simulink model "PQ_Control_LCL"  (R2023b)
settings: Solver=FixedStepAuto  StartTime=0.0  StopTime=10.0  RelTol=1e-3
InitFcn:
  | Initialization_for_PQ_Control_LCL;
values from neighbouring files (symbols this model uses):
  Fnom_Grid = 50    [Initialization_for_PQ_Control_LCL.m]
  Gain_for_ActiveDamping = 0.8    [VariablesDictionary_for_PQ_Control_LCL.sldd]
  Inom = Pnom/sqrt(3)/Unom_Grid    [Initialization_for_PQ_Control_LCL.m]
  Ki_Idq = Kp_Idq*2*pi*10    (= 157.913670417)    [Initialization_for_PQ_Control_LCL.m]
  Kp_Idq = L_grid*2*pi*2000    (= 2.51327412287)    [Initialization_for_PQ_Control_LCL.m]
  L_grid = 200e-6    (= 0.0002)    [Initialization_for_PQ_Control_LCL.m]
  Pnom = 220e3    (= 220000)    [Initialization_for_PQ_Control_LCL.m]
  Ts_Control = 62.5e-6    (= 6.25e-05)    [Initialization_for_PQ_Control_LCL.m]
  Udc_ref = 1500    [Initialization_for_PQ_Control_LCL.m]
  Unom_Phase = Unom_Grid/sqrt(3)    [Initialization_for_PQ_Control_LCL.m]
  Wp_compensation = 148.99    [VariablesDictionary_for_PQ_Control_LCL.sldd]
  Wz_compensation = 314.1592    [VariablesDictionary_for_PQ_Control_LCL.sldd]
libraries: LibraryForCodeGeneration x12
settings Model: DataDictionary=VariablesDictionary_for_PQ_Control_LCL.sldd  TunableVars=Inom,Ki_Idq,Kp_Idq,Udc_ref,Unom_Phase  TunableVarsStorageClass=Auto,Auto,Auto,Auto,Auto  TunableVarsTypeQualifier=,,,,  Creator=ZZY  LastModifiedBy=y
settings OptimizationCC: BlockReduction=off  DefaultParameterBehavior=Inlined  UseDivisionForNetSlopeComputation=on  DefaultUnderspecifiedDataType=single  ReuseModelBlockBuffer=off  ExpressionFolding=off  PassReuseOutputArgsAs=Individual arguments  ZeroExternalMemoryAtStartup=off  ZeroInternalMemoryAtStartup=off  EfficientFloat2IntCast=on  LifeSpan=inf  OptimizationLevel=level1  LabelGuidedReuse=on  EfficientTunableParamExpr=on
settings DebuggingCC: SignalInfNanChecking=warning  SignalRangeChecking=warning  ReadBeforeWriteMsg=EnableAllAsError  WriteAfterWriteMsg=EnableAllAsError  WriteAfterReadMsg=EnableAllAsError  IntegerOverflowMsg=error  ParameterPrecisionLossMsg=none  FixptConstUnderflowMsg=warning  FixptConstOverflowMsg=warning  FixptConstPrecisionLossMsg=warning  UnnecessaryDatatypeConvMsg=warning  UniqueDataStoreMsg=error  AssertControl=DisableAll  NonBusSignalsTreatedAsBus=error  SFInvalidInputDataAccessInChartInitDiag=error  SFTransitionOutsideNaturalParentDiag=error  SFUnreachableExecutionPathDiag=error  SFUndirectedBroadcastEventsDiag=error  IntegerSaturationMsg=error
settings HardwareCC: ProdBitPerChar=16  ProdBitPerInt=16  ProdBitPerPointer=32  ProdBitPerSizeT=32  ProdBitPerPtrDiffT=32  ProdLargestAtomicInteger=Integer  ProdLargestAtomicFloat=None  ProdWordSize=16  ProdHWDeviceType=Texas Instruments->C2000  TargetBitPerChar=16  TargetBitPerInt=16  TargetLargestAtomicInteger=Integer  TargetIntDivRoundTo=Zero  TargetEndianess=LittleEndian  TargetWordSize=16  TargetHWDeviceType=Texas Instruments->C2000
settings SFSimCC: CompileTimeRecursionLimit=0  EnableRuntimeRecursion=off  MATLABDynamicMemAlloc=off
settings RTWCC: Description=Embedded Coder  SystemTargetFile=ert.tlc  TemplateMakefile=ert_default_tmf  GenerateReport=on  Toolchain=MinGW64 | gmake (64-bit Windows)  BuildConfiguration=Faster Runs  IncludeHyperlinkInReport=on  LaunchReport=on  DataTypeReplacement=CDataTypesFixedWidth  GenerateTraceInfo=on  GenerateTraceReport=on  GenerateTraceReportSl=on  GenerateTraceReportSf=on  GenerateTraceReportEml=on  GenerateWebview=on  GenerateCodeReplacementReport=on  CheckMdlBeforeBuild=Warning
settings CodeAppCC: ForceParamTrailComments=on  IgnoreCustomStorageClasses=off  OperatorAnnotations=on  SimulinkDataObjDesc=on  SFDataObjDesc=on  MATLABFcnDesc=on  DefineNamingRule=UpperCase  InsertBlockDesc=on  StateflowObjectComments=on  MATLABSourceComments=on  InlinedPrmAccess=Macros  ReqsInCode=on
settings ERTTargetCC: TargetLangStandard=C99 (ISO)  GenerateSampleERTMain=on  CombineSignalStateStructs=on  GroupInternalDataByFunction=on  ParenthesesLevel=Standards  CastingMode=Standards  GenerateSharedConstants=off  ERTCustomFileTemplate=example_file_process.tlc  RateTransitionBlockCode=Function  PreserveExpressionOrder=on  PreserveIfCondition=on  ConvertIfToSwitch=off  SuppressUnreachableDefaultCases=off  EnableSignedLeftShifts=off  EnableSignedRightShifts=off  MaxIdInt64=INT64_MAX  MinIdInt64=INT64_MIN  MaxIdUint64=UINT64_MAX  MaxIdInt32=INT32_MAX  MinIdInt32=INT32_MIN  MaxIdUint32=UINT32_MAX  MaxIdInt16=INT16_MAX  MinIdInt16=INT16_MIN  MaxIdUint16=UINT16_MAX  MaxIdInt8=INT8_MAX  MinIdInt8=INT8_MIN  MaxIdUint8=UINT8_MAX

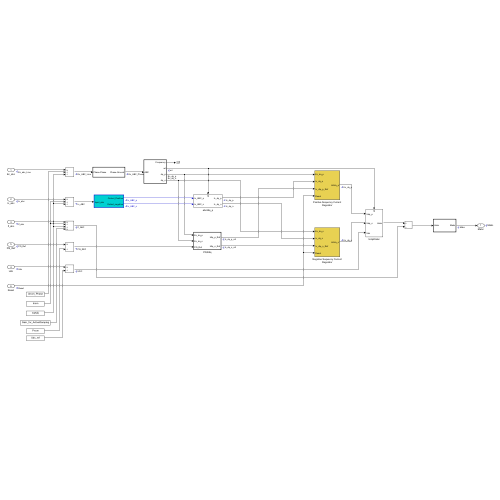
[thumbnail: Simulink's stored preview of the top-level diagram]
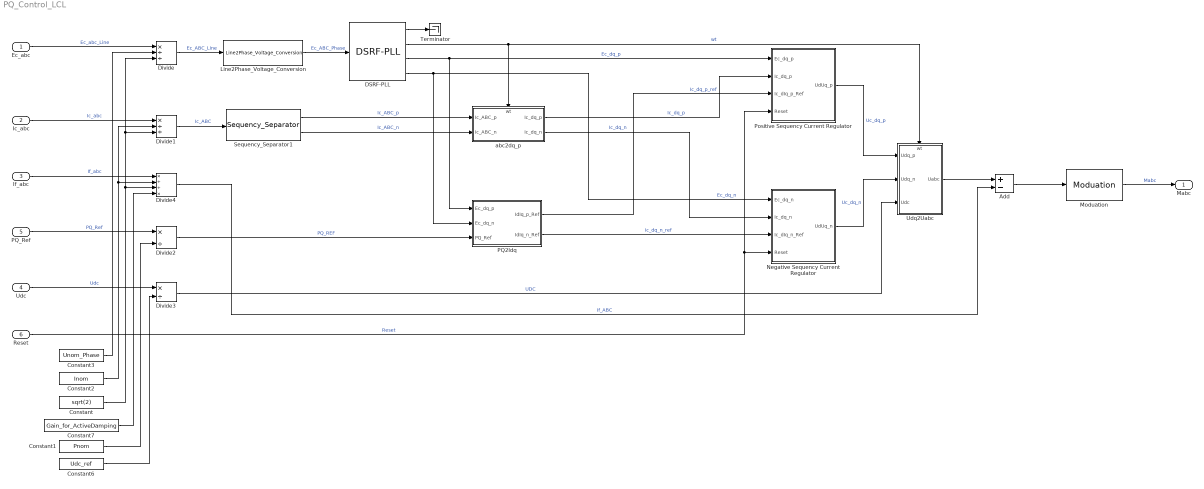
== system PQ_Control_LCL ==
  Ec_abc : Inport  OutDataTypeStr=single  PortDimensions=3
  Ic_abc : Inport  Port=2  OutDataTypeStr=single  PortDimensions=3
  If_abc : Inport  Port=3  OutDataTypeStr=single  PortDimensions=3
  Udc : Inport  Port=4  OutDataTypeStr=single
  PQ_Ref : Inport  Port=5  OutDataTypeStr=single
  Reset : Inport  Port=6  OutDataTypeStr=boolean
  Add : Sum  Inputs=+-
  Constant : Constant  Value=sqrt(2)  OutDataTypeStr=Inherit: Inherit via back propagation  SampleTime=-1
  Constant1 : Constant  Value=Pnom  OutDataTypeStr=Inherit: Inherit via back propagation  SampleTime=-1
  Constant2 : Constant  Value=Inom  OutDataTypeStr=Inherit: Inherit via back propagation  SampleTime=-1
  Constant3 : Constant  Value=Unom_Phase  OutDataTypeStr=Inherit: Inherit via back propagation  SampleTime=-1
  Constant6 : Constant  Value=Udc_ref  OutDataTypeStr=Inherit: Inherit via back propagation  SampleTime=-1
  Constant7 : Constant  Value=Gain_for_ActiveDamping  OutDataTypeStr=Inherit: Inherit via back propagation  SampleTime=-1
  DSRF-PLL : LibraryForCodeGeneration/DSRF-PLL  Ts=Ts_Control  Wc=2*pi*50*0.707  Wf=2*pi*50  Kp=2*pi*25*2*0.707  Ki=power(2*pi*25,2)
  Divide : Product  Inputs=*//  OutDataTypeStr=single
  Divide1 : Product  Inputs=*//  OutDataTypeStr=single
  Divide2 : Product  Inputs=*/  OutDataTypeStr=single
  Divide3 : Product  Inputs=*/  OutDataTypeStr=single
  Divide4 : Product  Inputs=*//*  OutDataTypeStr=single
  Line2Phase_Voltage_Conversion : LibraryForCodeGeneration/Line2Phase_Voltage_Conversion  SystemSampleTime=-1  VariantActivationTime=update diagram  AllowFlexibleInterface=on  Latency=0  AutoFrameSizeCalculation=off
  Moduation : LibraryForCodeGeneration/Moduation  Modulation=Modulation
  Negative Sequency Current Regulator : Subsystem
  PQ2Idq : Subsystem  TreatAsAtomicUnit=on
  Positive Sequency Current Regulator : Subsystem
  Sequency_Separator1 : LibraryForCodeGeneration/Sequency_Separator  SystemSampleTime=-1  VariantActivationTime=update diagram  AllowFlexibleInterface=on  Latency=0  AutoFrameSizeCalculation=off
  Terminator : Terminator
  Udq2Uabc : Subsystem
      settings: PortSchema="{\"entries\":[{\"content\":{\"sides\":[{\"content\":{\"connectorIds\":[\"In1\",\"In2\",\"In3\"]},\"type\":\"ConnectorPlacement.EquallySpacedRectSide\",\"uuid\":\"009786f4-728c-4160-b9bf-eaf0b5a05101\"},{\"content\":{\"connectorIds\":[\"Out1\"],\"side\":\"RIGHT\"},\"type\":\"ConnectorPlacement.EquallySpacedRectSide\",\"uuid\":\"2a94367a-5c57-4632-9573-ab089470159a\"},{\"content\":{\"connectorIds\":[\"In4\"],\"side\":\"TOP\"},\"type\":\"ConnectorPlacement.EquallySpacedRectSide\",\"uuid\":\"6906365b-3187-4c4b-97cf-c9dec4c5ef7c\"}]},\"type\":\"ConnectorPlacement.EquallySpacedConnector\",\"uuid\":\"96ca8566-a266-405c-817a-b47b433d51ed\"}],\"packageUris\":[\"http://schema.mathworks.com/mf0/Connector/R2020b\"],\"version\":\"1.0\"}"
  abc2dq_p : Subsystem
      settings: PortSchema="{\"entries\":[{\"content\":{\"sides\":[{\"content\":{\"connectorIds\":[\"In1\",\"In2\"]},\"type\":\"ConnectorPlacement.EquallySpacedRectSide\",\"uuid\":\"702c7fae-dbbb-427d-af19-afd468018ae6\"},{\"content\":{\"connectorIds\":[\"Out1\",\"Out2\"],\"side\":\"RIGHT\"},\"type\":\"ConnectorPlacement.EquallySpacedRectSide\",\"uuid\":\"d2ca5462-a446-46d8-bb73-1a455ffa959f\"},{\"content\":{\"connectorIds\":[\"In3\"],\"side\":\"TOP\"},\"type\":\"ConnectorPlacement.EquallySpacedRectSide\",\"uuid\":\"50bc6c44-424f-4342-960e-11540364fe97\"}]},\"type\":\"ConnectorPlacement.EquallySpacedConnector\",\"uuid\":\"f58cf64d-fe35-43f1-a031-7ee625a8bb1e\"}],\"packageUris\":[\"http://schema.mathworks.com/mf0/Connector/R2020b\"],\"version\":\"1.0\"}"
  Mabc : Outport  SignalName=Mabc  OutDataTypeStr=single  PortDimensions=3
      settings: MustResolveToSignalObject=on
  wires:
  Line2Phase_Voltage_Conversion/1 -> DSRF-PLL/1  "Ec_ABC_Phase"
  Divide2/1 -> PQ2Idq/3(PQ_Ref)  "PQ_REF"
  PQ_Ref/1 -> Divide2/1  "PQ_Ref"
  PQ2Idq/1(IdIq_p_Ref) -> Positive Sequency Current Regulator/3(Ic_dIq_p_Ref)  "Ic_dq_p_ref"
  abc2dq_p/2(Ic_dq_n) -> Negative Sequency Current Regulator/2(Ic_dq_n)  "Ic_dq_n"
  Positive Sequency Current Regulator/1(UdUq_p) -> Udq2Uabc/1(Udq_p)  "Uc_dq_p"
  Divide3/1 -> Udq2Uabc/3(Udc)  "UDC"
  DSRF-PLL/3 -> Positive Sequency Current Regulator/1(Ec_dq_p), PQ2Idq/1(Ec_dq_p)  "Ec_dq_p"
  Ec_abc/1 -> Divide/1  "Ec_abc_Line"
  abc2dq_p/1(Ic_dq_p) -> Positive Sequency Current Regulator/2(Ic_dq_p)  "Ic_dq_p"
  Divide1/1 -> Sequency_Separator1/1  "Ic_ABC"
  Ic_abc/1 -> Divide1/1  "Ic_abc"
  DSRF-PLL/4 -> Negative Sequency Current Regulator/1(Ec_dq_n), PQ2Idq/2(Ec_dq_n)  "Ec_dq_n"
  Divide/1 -> Line2Phase_Voltage_Conversion/1  "Ec_ABC_Line"
  Udc/1 -> Divide3/1  "Udc"
  PQ2Idq/2(IdIq_n_Ref) -> Negative Sequency Current Regulator/3(Ic_dIq_n_Ref)  "Ic_dq_n_ref"
  Constant3/1 -> Divide/2
  Constant/1 -> Divide4/3, Divide1/3, Divide/3
  Constant2/1 -> Divide4/2, Divide1/2
  Constant6/1 -> Divide3/2
  Reset/1 -> Positive Sequency Current Regulator/4(Reset), Negative Sequency Current Regulator/4(Reset)  "Reset"
  If_abc/1 -> Divide4/1  "If_abc"
  Divide4/1 -> Add/2  "If_ABC"
  DSRF-PLL/2 -> abc2dq_p/3(wt), Udq2Uabc/4(wt)  "wt"
  DSRF-PLL/1 -> Terminator/1
  Sequency_Separator1/2 -> abc2dq_p/2("Ic_ABC_n ")  "Ic_ABC_n"
  Sequency_Separator1/1 -> abc2dq_p/1("Ic_ABC_p ")  "Ic_ABC_p"
  Moduation/1 -> Mabc/1  "Mabc"
  Constant7/1 -> Divide4/4
  Add/1 -> Moduation/1
  Udq2Uabc/1(Uabc) -> Add/1
  Negative Sequency Current Regulator/1(UdUq_n) -> Udq2Uabc/2(Udq_n)  "Uc_dq_n"
  Constant1/1 -> Divide2/2

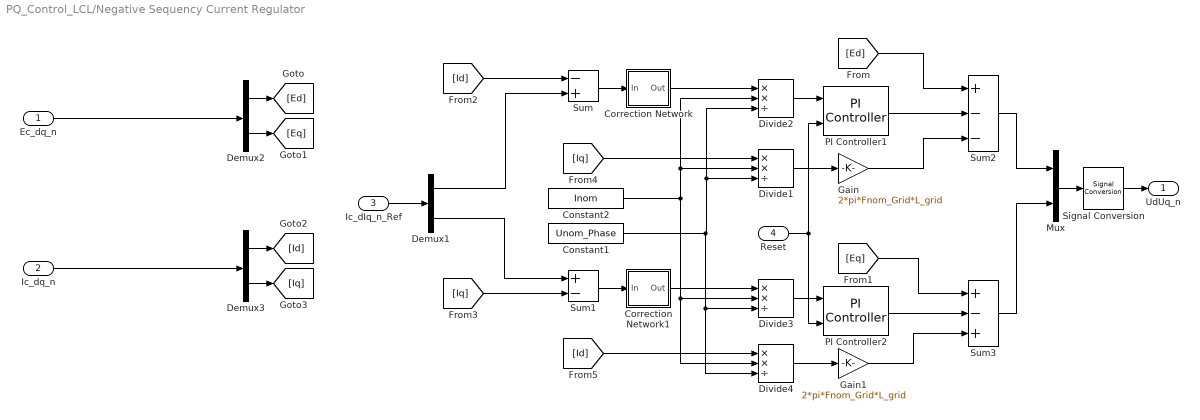
== system PQ_Control_LCL/Negative Sequency Current Regulator ==
  Ec_dq_n : Inport
  Ic_dq_n : Inport  Port=2
  Ic_dIq_n_Ref : Inport  Port=3
  Reset : Inport  Port=4  OutDataTypeStr=boolean
  Constant1 : Constant  Value=Unom_Phase  OutDataTypeStr=Inherit: Inherit via back propagation  SampleTime=-1
  Constant2 : Constant  Value=Inom  OutDataTypeStr=Inherit: Inherit via back propagation  SampleTime=-1
  Correction Network : Subsystem  mask{Ts=Ts_Control, p=Wp_compensation, z=Wz_compensation}
      mask prompts: Ts "Sampling Frequency:"; p "Pole Frequency:"; z "Zero Frequency:"
  Correction Network1 : Subsystem  mask{Ts=Ts_Control, p=Wp_compensation, z=Wz_compensation}
      mask prompts: Ts "Sampling Frequency:"; p "Pole Frequency:"; z "Zero Frequency:"
  Demux1 : Demux  Outputs=2
  Demux2 : Demux  Outputs=2
  Demux3 : Demux  Outputs=2
  Divide{1..4} (4 alike) : Product  Inputs=**/  OutDataTypeStr=single
  Gain : Gain  Gain=2*pi*Fnom_Grid*L_grid  ParamDataTypeStr=Inherit: Same as input
  Gain1 : Gain  Gain=2*pi*Fnom_Grid*L_grid  ParamDataTypeStr=Inherit: Same as input
  Mux : Mux  Inputs=2
  PI Controller1 : LibraryForCodeGeneration/PI Controller  Kp=Kp_Idq  Ki=Ki_Idq  Ts=Ts_Control  Max=2  Min=-2
  PI Controller2 : LibraryForCodeGeneration/PI Controller  Kp=Kp_Idq  Ki=Ki_Idq  Ts=Ts_Control  Max=2  Min=-2
  Signal Conversion : SignalConversion  OverrideOpt=off
  Sum : Sum  Inputs=-+  InputSameDT=on  SaturateOnIntegerOverflow=on  OutDataTypeStr=Inherit: Same as first input
  Sum1 : Sum  Inputs=+-  InputSameDT=on  SaturateOnIntegerOverflow=on  OutDataTypeStr=Inherit: Same as first input
  Sum2 : Sum  Inputs=+--  InputSameDT=on  SaturateOnIntegerOverflow=on  OutDataTypeStr=Inherit: Same as first input
  Sum3 : Sum  Inputs=+-+  InputSameDT=on  SaturateOnIntegerOverflow=on  OutDataTypeStr=Inherit: Same as first input
  UdUq_n : Outport
  wires:
  [Id] -> Divide4/1
  [Iq] -> Divide1/1
  [Iq] -> Sum1/2
  [Id] -> Sum/1
  Demux3/1 -> [Id]
  Demux3/2 -> [Iq]
  Demux1/2 -> Sum1/1
  Demux1/1 -> Sum/2
  [Eq] -> Sum3/1
  [Ed] -> Sum2/1
  Demux2/2 -> [Eq]
  Demux2/1 -> [Ed]
  Divide3/1 -> PI Controller2/1
  Sum/1 -> Correction Network/1(In)
  Mux/1 -> Signal Conversion/1
  Gain1/1 -> Sum3/3
  Gain/1 -> Sum2/3
  Ic_dIq_n_Ref/1 -> Demux1/1
  Sum2/1 -> Mux/1
  Sum1/1 -> Correction Network1/1(In)
  Divide2/1 -> PI Controller1/1
  Sum3/1 -> Mux/2
  Reset/1 -> PI Controller2/2, PI Controller1/2
  Divide1/1 -> Gain/1
  Divide4/1 -> Gain1/1
  Constant2/1 -> Divide1/2, Divide2/2, Divide4/2, Divide3/2
  Constant1/1 -> Divide3/3, Divide4/3, Divide1/3, Divide2/3
  PI Controller2/1 -> Sum3/2
  PI Controller1/1 -> Sum2/2
  Ec_dq_n/1 -> Demux2/1
  Signal Conversion/1 -> UdUq_n/1
  Ic_dq_n/1 -> Demux3/1
  Correction Network/1(Out) -> Divide2/1
  Correction Network1/1(Out) -> Divide3/1

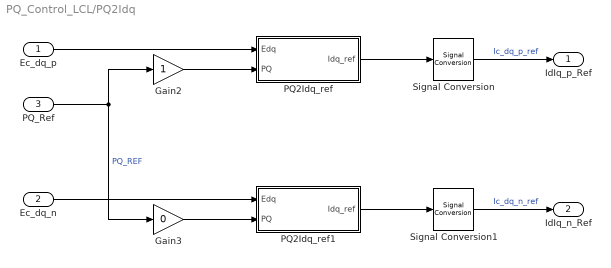
== system PQ_Control_LCL/PQ2Idq ==
  Ec_dq_p : Inport
  Ec_dq_n : Inport  Port=2
  PQ_Ref : Inport  Port=3
  Gain2 : Gain
  Gain3 : Gain  Gain=0
  PQ2Idq_ref : Subsystem  TreatAsAtomicUnit=on
  PQ2Idq_ref1 : Subsystem  TreatAsAtomicUnit=on
  Signal Conversion : SignalConversion  OverrideOpt=off
  Signal Conversion1 : SignalConversion  OverrideOpt=off
  IdIq_p_Ref : Outport
  IdIq_n_Ref : Outport  Port=2
  wires:
  Signal Conversion/1 -> IdIq_p_Ref/1  "Ic_dq_p_ref"
  Signal Conversion1/1 -> IdIq_n_Ref/1  "Ic_dq_n_ref"
  PQ_Ref/1 -> Gain2/1, Gain3/1  "PQ_REF"
  Ec_dq_p/1 -> PQ2Idq_ref/1(Edq)
  Gain2/1 -> PQ2Idq_ref/2(PQ)
  PQ2Idq_ref/1(Idq_ref) -> Signal Conversion/1
  Ec_dq_n/1 -> PQ2Idq_ref1/1(Edq)
  Gain3/1 -> PQ2Idq_ref1/2(PQ)
  PQ2Idq_ref1/1(Idq_ref) -> Signal Conversion1/1

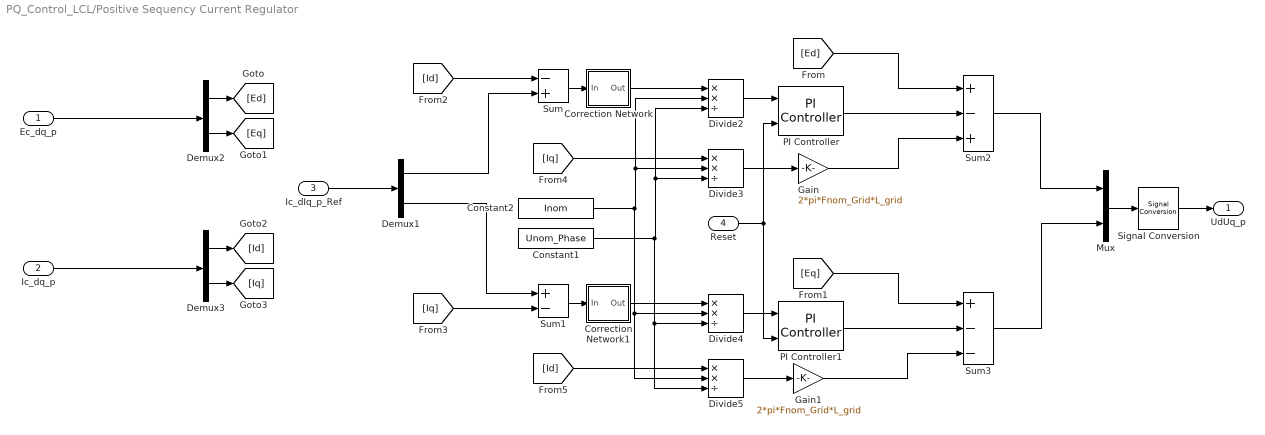
== system PQ_Control_LCL/Positive Sequency Current Regulator ==
  Ec_dq_p : Inport
  Ic_dq_p : Inport  Port=2
  Ic_dIq_p_Ref : Inport  Port=3
  Reset : Inport  Port=4  OutDataTypeStr=boolean
  Constant1 : Constant  Value=Unom_Phase  OutDataTypeStr=Inherit: Inherit via back propagation  SampleTime=-1
  Constant2 : Constant  Value=Inom  OutDataTypeStr=Inherit: Inherit via back propagation  SampleTime=-1
  Correction Network : Subsystem  mask{Ts=Ts_Control, p=Wp_compensation, z=Wz_compensation}
      mask prompts: Ts "Sampling Frequency:"; p "Pole Frequency:"; z "Zero Frequency:"
  Correction Network1 : Subsystem  mask{Ts=Ts_Control, p=Wp_compensation, z=Wz_compensation}
      mask prompts: Ts "Sampling Frequency:"; p "Pole Frequency:"; z "Zero Frequency:"
  Demux1 : Demux  Outputs=2
  Demux2 : Demux  Outputs=2
  Demux3 : Demux  Outputs=2
  Divide{2..5} (4 alike) : Product  Inputs=**/  OutDataTypeStr=single
  Gain : Gain  Gain=2*pi*Fnom_Grid*L_grid  ParamDataTypeStr=Inherit: Same as input
  Gain1 : Gain  Gain=2*pi*Fnom_Grid*L_grid  ParamDataTypeStr=Inherit: Same as input
  Mux : Mux  Inputs=2
  PI Controller : LibraryForCodeGeneration/PI Controller  Kp=Kp_Idq  Ki=Ki_Idq  Ts=Ts_Control  Max=2  Min=-2
  PI Controller1 : LibraryForCodeGeneration/PI Controller  Kp=Kp_Idq  Ki=Ki_Idq  Ts=Ts_Control  Max=2  Min=-2
  Signal Conversion : SignalConversion  OverrideOpt=off
  Sum : Sum  Inputs=-+  InputSameDT=on  SaturateOnIntegerOverflow=on  OutDataTypeStr=Inherit: Same as first input
  Sum1 : Sum  Inputs=+-  InputSameDT=on  SaturateOnIntegerOverflow=on  OutDataTypeStr=Inherit: Same as first input
  Sum2 : Sum  Inputs=+-+  InputSameDT=on  SaturateOnIntegerOverflow=on  OutDataTypeStr=Inherit: Same as first input
  Sum3 : Sum  Inputs=+--  InputSameDT=on  SaturateOnIntegerOverflow=on  OutDataTypeStr=Inherit: Same as first input
  UdUq_p : Outport
  wires:
  Sum3/1 -> Mux/2
  Sum1/1 -> Correction Network1/1(In)
  Sum2/1 -> Mux/1
  Ic_dIq_p_Ref/1 -> Demux1/1
  Divide3/1 -> Gain/1
  Divide5/1 -> Gain1/1
  Gain/1 -> Sum2/3
  Sum/1 -> Correction Network/1(In)
  Divide4/1 -> PI Controller1/1
  Demux2/1 -> [Ed]
  Demux2/2 -> [Eq]
  [Ed] -> Sum2/1
  Demux1/1 -> Sum/2
  Demux1/2 -> Sum1/1
  Demux3/2 -> [Iq]
  Demux3/1 -> [Id]
  [Id] -> Sum/1
  [Iq] -> Sum1/2
  [Iq] -> Divide3/1
  [Id] -> Divide5/1
  PI Controller/1 -> Sum2/2
  Divide2/1 -> PI Controller/1
  Reset/1 -> PI Controller1/2, PI Controller/2
  Constant2/1 -> Divide5/2, Divide4/2, Divide3/2, Divide2/2
  Constant1/1 -> Divide5/3, Divide4/3, Divide3/3, Divide2/3
  [Eq] -> Sum3/1
  PI Controller1/1 -> Sum3/2
  Gain1/1 -> Sum3/3
  Ec_dq_p/1 -> Demux2/1
  Mux/1 -> Signal Conversion/1
  Signal Conversion/1 -> UdUq_p/1
  Ic_dq_p/1 -> Demux3/1
  Correction Network/1(Out) -> Divide2/1
  Correction Network1/1(Out) -> Divide4/1

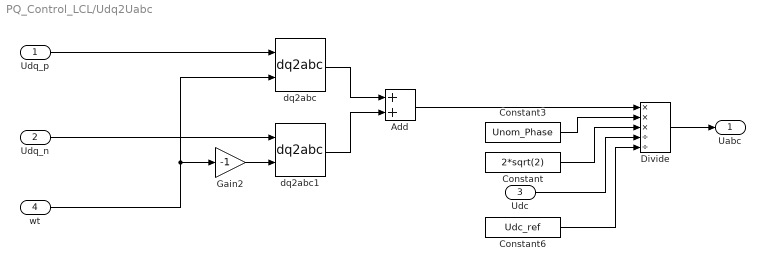
== system PQ_Control_LCL/Udq2Uabc ==
  Udq_p : Inport
  Udq_n : Inport  Port=2
  Udc : Inport  Port=3
  wt : Inport  Port=4
  Add : Sum
  Constant : Constant  Value=2*sqrt(2)  OutDataTypeStr=Inherit: Inherit via back propagation  SampleTime=-1
  Constant3 : Constant  Value=Unom_Phase  OutDataTypeStr=Inherit: Inherit via back propagation  SampleTime=-1
  Constant6 : Constant  Value=Udc_ref  OutDataTypeStr=Inherit: Inherit via back propagation  SampleTime=-1
  Divide : Product  Inputs=***//  OutDataTypeStr=single
  Gain2 : Gain  Gain=-1  ParamDataTypeStr=Inherit: Same as input
  dq2abc : LibraryForCodeGeneration/dq2abc  SystemSampleTime=-1  VariantActivationTime=update diagram  AllowFlexibleInterface=on  Latency=0  AutoFrameSizeCalculation=off
  dq2abc1 : LibraryForCodeGeneration/dq2abc  SystemSampleTime=-1  VariantActivationTime=update diagram  AllowFlexibleInterface=on  Latency=0  AutoFrameSizeCalculation=off
  Uabc : Outport
  wires:
  dq2abc1/1 -> Add/2
  wt/1 -> dq2abc/2, Gain2/1
  Gain2/1 -> dq2abc1/2
  Udq_p/1 -> dq2abc/1
  Udq_n/1 -> dq2abc1/1
  dq2abc/1 -> Add/1
  Constant6/1 -> Divide/5
  Constant/1 -> Divide/3
  Constant3/1 -> Divide/2
  Add/1 -> Divide/1
  Udc/1 -> Divide/4
  Divide/1 -> Uabc/1

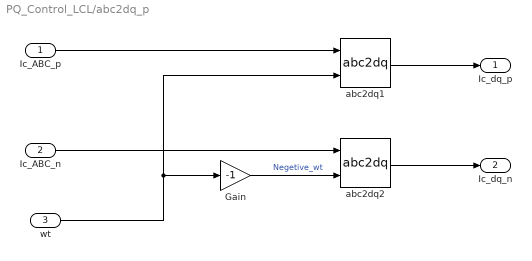
== system PQ_Control_LCL/abc2dq_p ==
  "Ic_ABC_p " : Inport
  "Ic_ABC_n " : Inport  Port=2
  wt : Inport  Port=3
  Gain : Gain  Gain=-1
  abc2dq1 : LibraryForCodeGeneration/abc2dq  SystemSampleTime=-1  VariantActivationTime=update diagram  AllowFlexibleInterface=on  Latency=0  AutoFrameSizeCalculation=off
  abc2dq2 : LibraryForCodeGeneration/abc2dq  SystemSampleTime=-1  VariantActivationTime=update diagram  AllowFlexibleInterface=on  Latency=0  AutoFrameSizeCalculation=off
  Ic_dq_p : Outport
  Ic_dq_n : Outport  Port=2
  wires:
  "Ic_ABC_p "/1 -> abc2dq1/1
  abc2dq1/1 -> Ic_dq_p/1
  Gain/1 -> abc2dq2/2  "Negetive_wt"
  "Ic_ABC_n "/1 -> abc2dq2/1
  abc2dq2/1 -> Ic_dq_n/1
  wt/1 -> abc2dq1/2, Gain/1

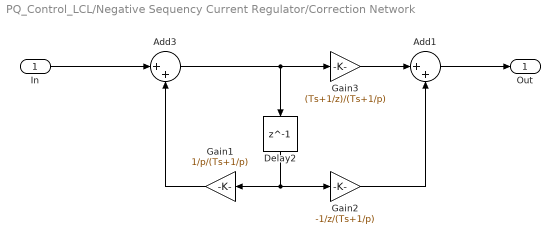
== system PQ_Control_LCL/Negative Sequency Current Regulator/Correction Network ==
  In : Inport
  Add1 : Sum  Inputs=|++
  Add3 : Sum  Inputs=|++
  Delay2 : Delay  DelayLength=1
  Gain1 : Gain  Gain=1/p/(Ts+1/p)
  Gain2 : Gain  Gain=-1/z/(Ts+1/p)
  Gain3 : Gain  Gain=(Ts+1/z)/(Ts+1/p)
  Out : Outport
  wires:
  Gain1/1 -> Add3/2
  Add3/1 -> Gain3/1, Delay2/1
  In/1 -> Add3/1
  Delay2/1 -> Gain1/1, Gain2/1
  Gain2/1 -> Add1/2
  Gain3/1 -> Add1/1
  Add1/1 -> Out/1

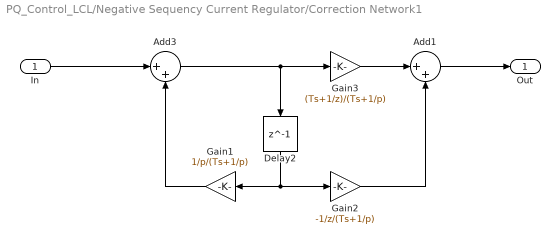
== system PQ_Control_LCL/Negative Sequency Current Regulator/Correction Network1 ==
  In : Inport
  Add1 : Sum  Inputs=|++
  Add3 : Sum  Inputs=|++
  Delay2 : Delay  DelayLength=1
  Gain1 : Gain  Gain=1/p/(Ts+1/p)
  Gain2 : Gain  Gain=-1/z/(Ts+1/p)
  Gain3 : Gain  Gain=(Ts+1/z)/(Ts+1/p)
  Out : Outport
  wires:
  Gain1/1 -> Add3/2
  Add3/1 -> Gain3/1, Delay2/1
  In/1 -> Add3/1
  Delay2/1 -> Gain1/1, Gain2/1
  Gain2/1 -> Add1/2
  Gain3/1 -> Add1/1
  Add1/1 -> Out/1

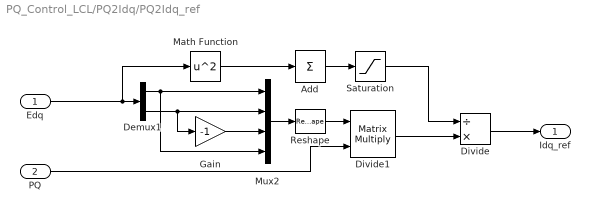
== system PQ_Control_LCL/PQ2Idq/PQ2Idq_ref ==
  Edq : Inport
  PQ : Inport  Port=2
  Add : Sum  Inputs=+
  Demux1 : Demux  Outputs=2
  Divide : Product  Inputs=/*
  Divide1 : Product  Inputs=**  Multiplication=Matrix(*)
  Gain : Gain  Gain=-1
  Math Function : Math  Operator=square  OutMin=[0.5]  OutMax=[2]
  Mux2 : Mux
  Reshape : Reshape  OutputDimensionality=Customize  OutputDimensions=[2,2]
  Saturation : Saturate  UpperLimit=1.5  LowerLimit=0.1
  Idq_ref : Outport
  wires:
  Demux1/2 -> Mux2/2, Gain/1
  Divide1/1 -> Divide/2
  Edq/1 -> Math Function/1, Demux1/1
  Mux2/1 -> Reshape/1
  Add/1 -> Saturation/1
  Math Function/1 -> Add/1
  Demux1/1 -> Mux2/4, Mux2/1
  Saturation/1 -> Divide/1
  Divide/1 -> Idq_ref/1
  Reshape/1 -> Divide1/1
  Gain/1 -> Mux2/3
  PQ/1 -> Divide1/2

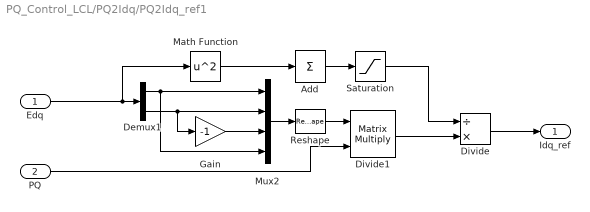
== system PQ_Control_LCL/PQ2Idq/PQ2Idq_ref1 ==
  Edq : Inport
  PQ : Inport  Port=2
  Add : Sum  Inputs=+
  Demux1 : Demux  Outputs=2
  Divide : Product  Inputs=/*
  Divide1 : Product  Inputs=**  Multiplication=Matrix(*)
  Gain : Gain  Gain=-1
  Math Function : Math  Operator=square  OutMin=[0.5]  OutMax=[2]
  Mux2 : Mux
  Reshape : Reshape  OutputDimensionality=Customize  OutputDimensions=[2,2]
  Saturation : Saturate  UpperLimit=1.5  LowerLimit=0.1
  Idq_ref : Outport
  wires:
  Demux1/2 -> Mux2/2, Gain/1
  Divide1/1 -> Divide/2
  Edq/1 -> Math Function/1, Demux1/1
  Mux2/1 -> Reshape/1
  Add/1 -> Saturation/1
  Math Function/1 -> Add/1
  Demux1/1 -> Mux2/4, Mux2/1
  Saturation/1 -> Divide/1
  Divide/1 -> Idq_ref/1
  Reshape/1 -> Divide1/1
  Gain/1 -> Mux2/3
  PQ/1 -> Divide1/2

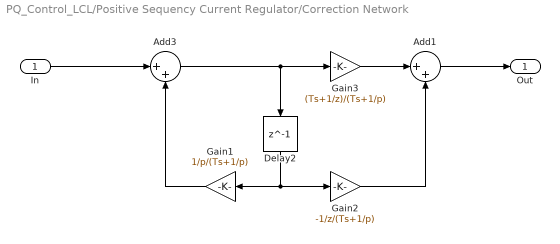
== system PQ_Control_LCL/Positive Sequency Current Regulator/Correction Network ==
  In : Inport
  Add1 : Sum  Inputs=|++
  Add3 : Sum  Inputs=|++
  Delay2 : Delay  DelayLength=1
  Gain1 : Gain  Gain=1/p/(Ts+1/p)
  Gain2 : Gain  Gain=-1/z/(Ts+1/p)
  Gain3 : Gain  Gain=(Ts+1/z)/(Ts+1/p)
  Out : Outport
  wires:
  Gain1/1 -> Add3/2
  Add3/1 -> Gain3/1, Delay2/1
  In/1 -> Add3/1
  Delay2/1 -> Gain1/1, Gain2/1
  Gain2/1 -> Add1/2
  Gain3/1 -> Add1/1
  Add1/1 -> Out/1

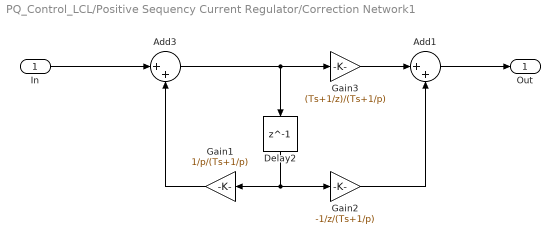
== system PQ_Control_LCL/Positive Sequency Current Regulator/Correction Network1 ==
  In : Inport
  Add1 : Sum  Inputs=|++
  Add3 : Sum  Inputs=|++
  Delay2 : Delay  DelayLength=1
  Gain1 : Gain  Gain=1/p/(Ts+1/p)
  Gain2 : Gain  Gain=-1/z/(Ts+1/p)
  Gain3 : Gain  Gain=(Ts+1/z)/(Ts+1/p)
  Out : Outport
  wires:
  Gain1/1 -> Add3/2
  Add3/1 -> Gain3/1, Delay2/1
  In/1 -> Add3/1
  Delay2/1 -> Gain1/1, Gain2/1
  Gain2/1 -> Add1/2
  Gain3/1 -> Add1/1
  Add1/1 -> Out/1
